simulink model "non_linear_simulation_v2"  (R2020a)
settings: Solver=ode4  StartTime=0.0  StopTime=inf  FixedStep=0.01  RelTol=1e-3
InitFcn:
  | run('initialize_system.m')
values from neighbouring files (symbols this model uses):
  Ac = [d_f1_dth,d_f1_dyw,d_f1_dw_th,d_f1_dw_yw ... (first row only)    [linearize_heli.m]
  Bc = [d_f1_Vmp,d_f1_Vmy ... (first row only)    [linearize_heli.m]
  Cc = [1,0,0,0;0,1,0,0]    [linearize_heli.m]
  Q = diag([5e1,7e1,8e1,6e1])    [initialize_system.m]
  R = diag([0.1,0.1])    [initialize_system.m]
  th_op = -30*pi/180    (= -0.523598775598)    [initialize_system.m]
  Vmp_op = (Kyy*m_heli*g*cos(th_op)*l_cm) / (Kyy*Kpp - Kyp*Kpy)    [initialize_system.m]
  Vmy_op = (Kyp*Vmp_op) / (Kyy)    [initialize_system.m]
  w_th_op = 0    [initialize_system.m]
  w_yw_op = 0    [initialize_system.m]
  yw_op = pi/2    (= 1.57079632679)    [initialize_system.m]
undefined symbols (not defined in the file or in its folder): L, P0
libraries: realtime_pacer_lib x1, dspsigops x1
(part 1 of 2)
settings Model: Creator=engen  LastModifiedBy=engen

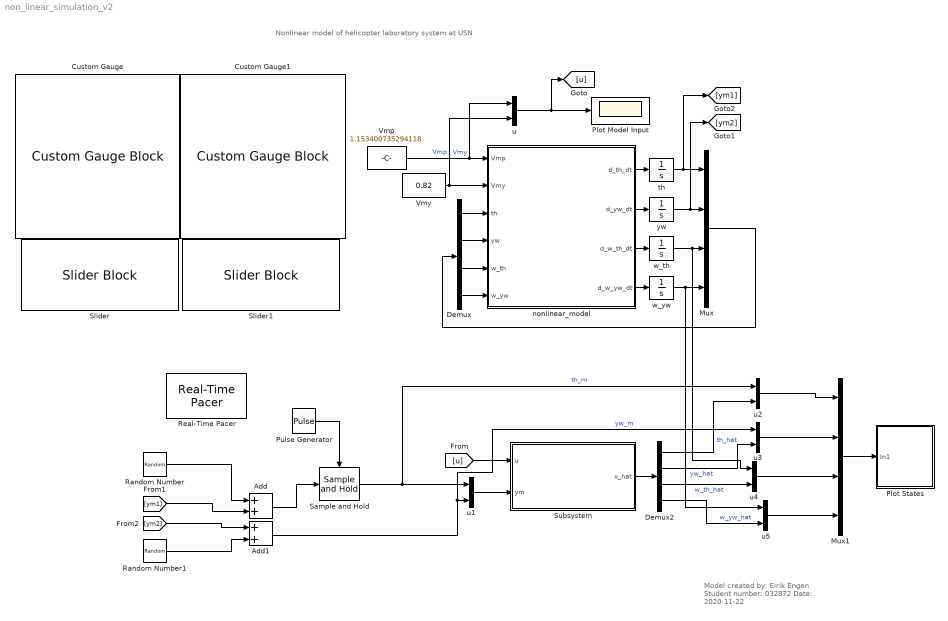
== system non_linear_simulation_v2 ==
  note: Model created by: Eirik Engen
      | Student number: 032872
      | Date: 2020-11-22
  note: Nonlinear model of helicopter laboratory system at USN
  Add : Sum
  Add1 : Sum
  Custom Gauge : CustomGaugeBlock  NeedleImage=data:image/svg+xml;base64,PD94bWwgdmVyc2lvbj0iMS4wIiBlbmNvZGluZz0idXRmLTgiPz4KPCEtLSBHZW5lcmF0b3I6IEFkb2JlIElsbHVzdHJhdG9yIDE5LjIuMSwgU1ZHIEV4cG9ydCBQbHVnLUluIC4gU1ZHIFZlcnNpb246IDYuMDAgQnVpbGQgMCkgIC0tPgo8c3ZnIHZlcnNpb249IjEuMSIgeG1sbnM9Imh0dHA6Ly93d3cudzMub3JnLzIwMDAvc3ZnIiB4bWxuczp4bGluaz0iaHR0cDovL3d3dy53My5vcmcvMTk5OS94bGluayIgeD0iMHB4IiB5PSIwcHgiCgkgdmlld0JveD0iMCAwIDIwMCA1MCIgc3R5bGU9ImVuYWJsZS1iYWNrZ3JvdW5kOm5ldyAw ...(+9940 chars)  NeedleXPos=0.39170480046297973  NeedleYPos=0.48297683576593553  NeedleHeight=0.10490569201603189  NeedleWidth=0.17282438115971863  NeedleInitialRotation=-59.94322499147643  BackgroundImage=data:image/svg+xml;base64,PD94bWwgdmVyc2lvbj0iMS4wIiBlbmNvZGluZz0iVVRGLTgiIHN0YW5kYWxvbmU9Im5vIj8+CjwhLS0gR2VuZXJhdG9yOiBBZG9iZSBJbGx1c3RyYXRvciAxOS4yLjEsIFNWRyBFeHBvcnQgUGx1Zy1JbiAuIFNWRyBWZXJzaW9uOiA2LjAwIEJ1aWxkIDApICAtLT4KCjxzdmcKICAgeG1sbnM6ZGM9Imh0dHA6Ly9wdXJsLm9yZy9kYy9lbGVtZW50cy8xLjEvIgogICB4bWxuczpjYz0iaHR0cDovL2NyZWF0aXZlY29tbW9ucy5vcmcvbnMjIgogICB4bWxuczpyZGY9Imh0dHA6Ly93d3cudzMub3JnLzE5OTkvMDIvMjItcmRmLXN5bnRh ...(+9660 chars)  GaugeMax=5  GaugeArcDefined=true  GaugeArcRadius=0.1228402170665963  GaugeArcStrokeWidth=0.03592322137076784  GaugeArcRotation=240.5385250290321  GaugeArcRatio=0.8333333333333  GaugeArcTransparency=0  ValueArcColor=#1759b0  GaugeTickColor=#faf5c8  ScaleColorsJSON="[{\"Min\":0,\"Max\":1.1,\"Color\":[1,1,0]},{\"Min\":1.1,\"Max\":1.4,\"Color\":[0,1,0]},{\"Min\":1.4,\"Max\":5,\"Color\":[1,1,0]}]"  fixedAspectRatio=on  IsLinearGauge=false  GaugeTrackLeft=0.35  GaugeTrackTop=0.35  GaugeTrackHeight=0.1  GaugeTrackWidth=0.3  GaugeTrackRotation=0
  Custom Gauge1 : CustomGaugeBlock  NeedleImage=data:image/svg+xml;base64,PD94bWwgdmVyc2lvbj0iMS4wIiBlbmNvZGluZz0idXRmLTgiPz4KPCEtLSBHZW5lcmF0b3I6IEFkb2JlIElsbHVzdHJhdG9yIDE5LjIuMSwgU1ZHIEV4cG9ydCBQbHVnLUluIC4gU1ZHIFZlcnNpb246IDYuMDAgQnVpbGQgMCkgIC0tPgo8c3ZnIHZlcnNpb249IjEuMSIgeG1sbnM9Imh0dHA6Ly93d3cudzMub3JnLzIwMDAvc3ZnIiB4bWxuczp4bGluaz0iaHR0cDovL3d3dy53My5vcmcvMTk5OS94bGluayIgeD0iMHB4IiB5PSIwcHgiCgkgdmlld0JveD0iMCAwIDIwMCA1MCIgc3R5bGU9ImVuYWJsZS1iYWNrZ3JvdW5kOm5ldyAw ...(+9940 chars)  NeedleXPos=0.39170480046297973  NeedleYPos=0.48297683576593553  NeedleHeight=0.10490569201603189  NeedleWidth=0.17282438115971863  NeedleInitialRotation=-59.94322499147643  BackgroundImage=data:image/svg+xml;base64,PD94bWwgdmVyc2lvbj0iMS4wIiBlbmNvZGluZz0iVVRGLTgiIHN0YW5kYWxvbmU9Im5vIj8+CjwhLS0gR2VuZXJhdG9yOiBBZG9iZSBJbGx1c3RyYXRvciAxOS4yLjEsIFNWRyBFeHBvcnQgUGx1Zy1JbiAuIFNWRyBWZXJzaW9uOiA2LjAwIEJ1aWxkIDApICAtLT4KCjxzdmcKICAgeG1sbnM6ZGM9Imh0dHA6Ly9wdXJsLm9yZy9kYy9lbGVtZW50cy8xLjEvIgogICB4bWxuczpjYz0iaHR0cDovL2NyZWF0aXZlY29tbW9ucy5vcmcvbnMjIgogICB4bWxuczpyZGY9Imh0dHA6Ly93d3cudzMub3JnLzE5OTkvMDIvMjItcmRmLXN5bnRh ...(+9660 chars)  GaugeMax=5  GaugeArcDefined=true  GaugeArcRadius=0.1228402170665963  GaugeArcStrokeWidth=0.03592322137076784  GaugeArcRotation=240.5385250290321  GaugeArcRatio=0.8333333333333  GaugeArcTransparency=0  ValueArcColor=#1759b0  GaugeTickColor=#faf5c8  ScaleColorsJSON="[{\"Min\":0,\"Max\":0.4,\"Color\":[1,1,0]},{\"Min\":0.4,\"Max\":1.3,\"Color\":[0,1,0]},{\"Min\":1.3,\"Max\":5,\"Color\":[1,1,0]}]"  fixedAspectRatio=on  IsLinearGauge=false  GaugeTrackLeft=0.35  GaugeTrackTop=0.35  GaugeTrackHeight=0.1  GaugeTrackWidth=0.3  GaugeTrackRotation=0
  Demux : Demux
  Demux2 : Demux
  Mux : Mux
  Mux1 : Mux
  Plot Model Input : Scope
  Plot States : Subsystem
  Pulse Generator : DiscretePulseGenerator  PulseType=Time based  Period=0.5  PulseWidth=50
  Random Number : RandomNumber  Variance=1e-5  Seed=0.01  SampleTime=0.1
  Random Number1 : RandomNumber  Variance=1e-5  SampleTime=0.1
  Real-Time Pacer : realtime_pacer_lib/Real-Time Pacer  simTimePerRealTime=1
      settings: SourceProductName=Real-Time Pacer
  Sample and Hold : dspsigops/Sample and Hold  trig=Rising edge  initCond=0  latchinput=off
  Slider : SliderBlock  ScaleMax=1.5
  Slider1 : SliderBlock  ScaleMax=1.5
  Subsystem : Subsystem
  Vmp : Constant  Value=1.153400735294118  SampleTime=-1
  Vmy : Constant  Value=0.82  SampleTime=-1
  nonlinear_model : MATLAB Function  TreatAsAtomicUnit=on
  th : Integrator  InitialCondition=-45*pi/180  LimitOutput=on  UpperSaturationLimit=45*pi/180  LowerSaturationLimit=-45*pi/180  ContinuousStateAttributes='th'
  u{,1..5} (6 alike) : Mux  Inputs=2
  w_th : Integrator  ContinuousStateAttributes='w_th'
  w_yw : Integrator  ContinuousStateAttributes='w_yw'
  yw : Integrator  LimitOutput=on  UpperSaturationLimit=180*pi/180  LowerSaturationLimit=0  ContinuousStateAttributes='yw'
  wires:
  Vmp/1 -> u/1, nonlinear_model/1(Vmp)  "Vmp"
  Vmy/1 -> u/2, nonlinear_model/2(Vmy)  "Vmy"
  nonlinear_model/1(d_th_dt) -> th/1
  nonlinear_model/2(d_yw_dt) -> yw/1
  nonlinear_model/3(d_w_th_dt) -> w_th/1
  nonlinear_model/4(d_w_yw_dt) -> w_yw/1
  th/1 -> [ym1], Mux/1
  yw/1 -> [ym2], Mux/2
  w_th/1 -> u4/1, Mux/3
  w_yw/1 -> u5/1, Mux/4
  Mux/1 -> Demux/1
  Demux/1 -> nonlinear_model/3(th)
  Demux/2 -> nonlinear_model/4(yw)
  Demux/3 -> nonlinear_model/5(w_th)
  Demux/4 -> nonlinear_model/6(w_yw)
  u/1 -> [u], Plot Model Input/1
  [u] -> Subsystem/1(u)
  u1/1 -> Subsystem/2(ym)
  Random Number/1 -> Add/1
  [ym1] -> Add/2
  Random Number1/1 -> Add1/2
  [ym2] -> Add1/1
  Add1/1 -> u3/1, u1/2  "yw_m"
  Subsystem/1(x_hat) -> Demux2/1
  Mux1/1 -> Plot States/1(In1)
  u2/1 -> Mux1/1
  u3/1 -> Mux1/2
  Demux2/1 -> u2/2  "th_hat"
  Demux2/2 -> u3/2  "yw_hat"
  u5/1 -> Mux1/4
  u4/1 -> Mux1/3
  Add/1 -> Sample and Hold/1
  Sample and Hold/1 -> u2/1, u1/1  "th_m"
  Pulse Generator/1 -> Sample and Hold/Trigger
  Demux2/4 -> u5/2  "w_yw_hat"
  Demux2/3 -> u4/2  "w_th_hat"

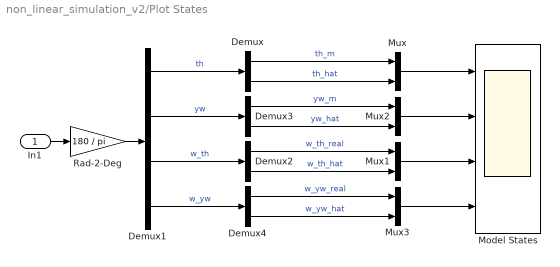
== system non_linear_simulation_v2/Plot States ==
  In1 : Inport
  Demux{,2..4} (4 alike) : Demux  Outputs=2
  Demux1 : Demux
  Model States : Scope  NumInputPorts=4
  Mux{,1..3} (4 alike) : Mux  Inputs=2
  Rad-2-Deg : Gain  Gain=180 / pi
  wires:
  In1/1 -> Rad-2-Deg/1
  Rad-2-Deg/1 -> Demux1/1
  Demux/1 -> Mux/1  "th_m"
  Demux/2 -> Mux/2  "th_hat"
  Demux3/1 -> Mux2/1  "yw_m"
  Demux3/2 -> Mux2/2  "yw_hat"
  Demux2/1 -> Mux1/1  "w_th_real"
  Demux2/2 -> Mux1/2  "w_th_hat"
  Demux4/1 -> Mux3/1  "w_yw_real"
  Demux4/2 -> Mux3/2  "w_yw_hat"
  Demux1/1 -> Demux/1  "th"
  Demux1/2 -> Demux3/1  "yw"
  Demux1/3 -> Demux2/1  "w_th"
  Demux1/4 -> Demux4/1  "w_yw"
  Mux/1 -> Model States/1
  Mux2/1 -> Model States/2
  Mux1/1 -> Model States/3
  Mux3/1 -> Model States/4

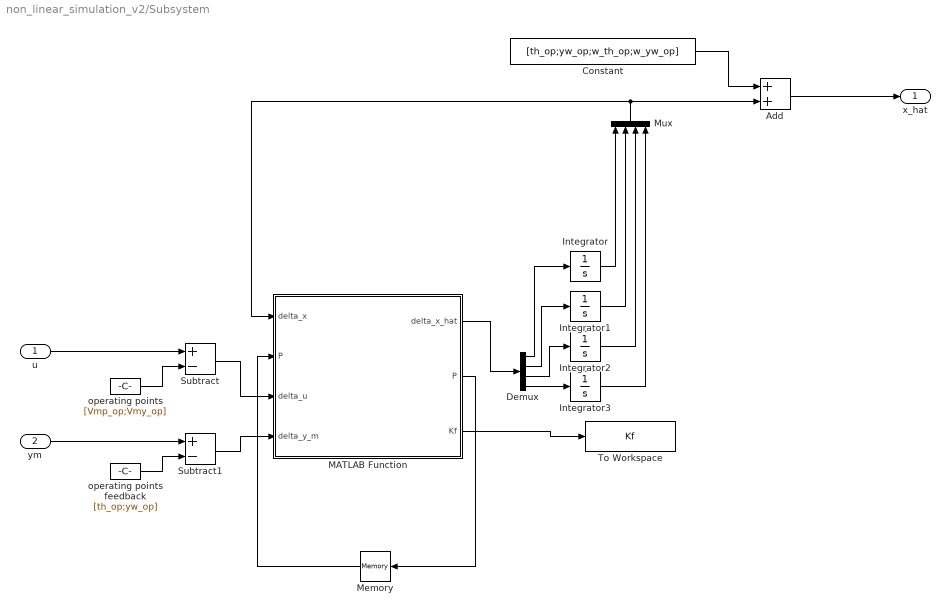
== system non_linear_simulation_v2/Subsystem ==
  u : Inport
  ym : Inport  Port=2
  Add : Sum
  Constant : Constant  Value=[th_op;yw_op;w_th_op;w_yw_op]
  Demux : Demux
  Integrator{,1..3} (4 alike) : Integrator
  MATLAB Function : MATLAB Function  TreatAsAtomicUnit=on
  Memory : Memory  InitialCondition=P0
  Mux : Mux
  Subtract : Sum  Inputs=+-
  Subtract1 : Sum  Inputs=+-
  To Workspace : ToWorkspace  VariableName=Kf  SaveFormat=Structure  SampleTime=-1
      settings: Save2DSignal=2-D array (concatenate along first dimension)
  operating points : Constant  Value=[Vmp_op;Vmy_op]
  operating points feedback : Constant  Value=[th_op;yw_op]
  x_hat : Outport
  wires:
  MATLAB Function/1(delta_x_hat) -> Demux/1
  u/1 -> Subtract/1
  operating points/1 -> Subtract/2
  Subtract/1 -> MATLAB Function/3(delta_u)
  Mux/1 -> MATLAB Function/1(delta_x), Add/2
  Demux/1 -> Integrator/1
  Demux/2 -> Integrator1/1
  Demux/3 -> Integrator2/1
  Demux/4 -> Integrator3/1
  Integrator/1 -> Mux/1
  Integrator1/1 -> Mux/2
  Integrator2/1 -> Mux/3
  Integrator3/1 -> Mux/4
  Subtract1/1 -> MATLAB Function/4(delta_y_m)
  ym/1 -> Subtract1/1
  operating points feedback/1 -> Subtract1/2
  Constant/1 -> Add/1
  Add/1 -> x_hat/1
  MATLAB Function/2(P) -> Memory/1
  Memory/1 -> MATLAB Function/2("P ")
  MATLAB Function/3(Kf) -> To Workspace/1

== matlab function non_linear_simulation_v2/Subsystem/MATLAB Function ==
  data: delta_x input; P input; delta_u input; delta_x_hat output size=4; delta_y_m input; Ac parameter; Bc parameter; Cc parameter; L parameter; P output; R parameter; Q parameter; Kf output
function [delta_x_hat, P, Kf] = linear_state_observer(delta_x,P, delta_u,delta_y_m,Ac,Bc,Cc,L,R, Q)
    
    % Compute apriori state covariance
    P = Ac*P*Ac' + Q;
    % Kalman gain
    Kf = (P*Cc')/(Cc*P*Cc'+R);
    %apriori state
    delta_x_hat = Ac*delta_x + Bc*delta_u;
    %estimated output    
    y_hat = Cc*delta_x;
    % aposteriori state
    delta_x_hat = delta_x_hat + Bc*delta_u + Kf*(delta_y_m - y_hat);
    % Update state covariance
    P = (eye(size(Kf*Cc)) - Kf*Cc)*P*(eye(size(Kf*Cc))-Kf*Cc)' + Kf*R*Kf';
